simulink model "COMPTORQUE_Amato"  (R2018b)
settings: Solver=VariableStepAuto  StartTime=0.0  StopTime=10  RelTol=1e-3
values from neighbouring files (symbols this model uses):
  cond_init = [x1,x2,x3,x4,x5,x6]'    [Init.m]    (also in WS_regressor.mat = [0.523598775598 2.09439510239 -1.0471975512 1.57079632679 1.)
  Law = [kp, kd]    [Init.m]    (also in LAUNCH_Backstepping.m = [lambda, kd]; LAUNCH_Backstepping_adapt.m; LAUNCH_CToque.m; WS_regressor.mat = [500 50])
  param = param'    [Init.m]    (also in WS_regressor.mat = [1 1 1 1 1 1 0 1 1 1 3 3 ... (14 elements, 7x2)])
  pulsazione_circolare = 1    [Init.m]    (also in WS_regressor.mat)
  x0 = -1.5    [Init.m]    (also in WS_regressor.mat)
  y0 = 2    [Init.m]    (also in WS_regressor.mat)
undefined symbols (not defined in the file or in its folder): A_circolare
libraries: simulink x1
settings Model: Creator=AmatoPi  LastModifiedBy=Utente

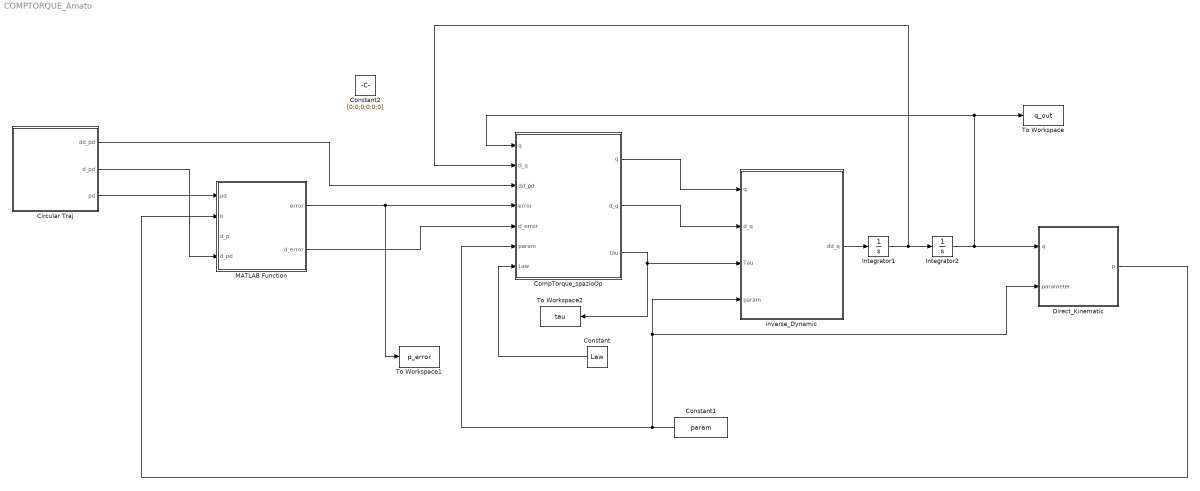
== system COMPTORQUE_Amato ==
  Circular Traj : Subsystem
  CompTorque_spazioOp : MATLAB Function  TreatAsAtomicUnit=on
  Constant : Constant  Value=Law
  Constant1 : Constant  Value=param
  Constant2 : Constant  Value=[0;0;0;0;0;0]
  Direct_Kinematic : MATLAB Function  TreatAsAtomicUnit=on
  Integrator1 : Integrator  InitialCondition=[0;0;0;0;0;0]
  Integrator2 : Integrator  InitialCondition=cond_init
  MATLAB Function : MATLAB Function  TreatAsAtomicUnit=on
  To Workspace : ToWorkspace  VariableName=q_out  SaveFormat=Structure With Time  SampleTime=-1
  To Workspace1 : ToWorkspace  VariableName=p_error  SaveFormat=Structure With Time  SampleTime=-1
  To Workspace2 : ToWorkspace  VariableName=tau  SaveFormat=Structure With Time  SampleTime=-1
  inverse_Dynamic : MATLAB Function  TreatAsAtomicUnit=on
  wires:
  CompTorque_spazioOp/2(d_q) -> inverse_Dynamic/2(d_q)
  CompTorque_spazioOp/1(q) -> inverse_Dynamic/1(q)
  inverse_Dynamic/1(dd_q) -> Integrator1/1
  Integrator1/1 -> CompTorque_spazioOp/2("d_q "), Integrator2/1
  Integrator2/1 -> CompTorque_spazioOp/1("q "), To Workspace/1, Direct_Kinematic/1(q)
  Constant/1 -> CompTorque_spazioOp/7(Law)
  Constant1/1 -> Direct_Kinematic/2(parameter), inverse_Dynamic/4(param), CompTorque_spazioOp/6(param)
  Circular Traj/3(pd) -> MATLAB Function/1(pd)
  Direct_Kinematic/1(p) -> MATLAB Function/2(p)
  MATLAB Function/1(error) -> To Workspace1/1, CompTorque_spazioOp/4(error)
  CompTorque_spazioOp/3(tau) -> To Workspace2/1, inverse_Dynamic/3(Tau)
  MATLAB Function/2(d_error) -> CompTorque_spazioOp/5(d_error)
  Circular Traj/2(d_pd) -> MATLAB Function/4(d_pd)
  Circular Traj/1(dd_pd) -> CompTorque_spazioOp/3(dd_pd)

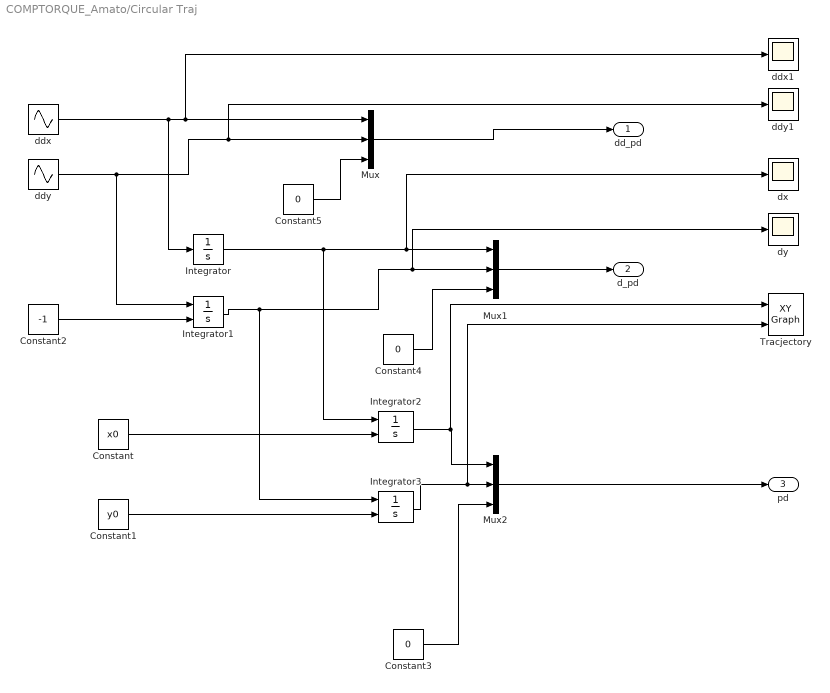
== system COMPTORQUE_Amato/Circular Traj ==
  Constant : Constant  Value=x0
  Constant1 : Constant  Value=y0
  Constant2 : Constant  Value=-1
  Constant3 : Constant  Value=0
  Constant4 : Constant  Value=0
  Constant5 : Constant  Value=0
  Integrator : Integrator
  Integrator1 : Integrator  InitialConditionSource=external
  Integrator2 : Integrator  InitialConditionSource=external
  Integrator3 : Integrator  InitialConditionSource=external
  Mux : Mux  Inputs=3
  Mux1 : Mux  Inputs=3
  Mux2 : Mux  Inputs=3
  Tracjectory : simulink/Sinks/XY Graph  xmin=xL  xmax=xR  ymin=yD  ymax=yU  st=-1
  ddx : Sin  Amplitude=A_circolare  Frequency=pulsazione_circolare  Phase=pi/2  SampleTime=0
  ddx1 : Scope
  ddy : Sin  Amplitude=A_circolare  Frequency=pulsazione_circolare  SampleTime=0
  ddy1 : Scope
  dx : Scope
  dy : Scope
  dd_pd : Outport
  d_pd : Outport  Port=2
  pd : Outport  Port=3
  wires:
  Mux/1 -> dd_pd/1
  ddx/1 -> Integrator/1, ddx1/1, Mux/1
  ddy/1 -> ddy1/1, Mux/2, Integrator1/1
  Mux1/1 -> d_pd/1
  Integrator2/1 -> Tracjectory/1, Mux2/1
  Mux2/1 -> pd/1
  Integrator/1 -> Integrator2/1, dx/1, Mux1/1
  Integrator3/1 -> Tracjectory/2, Mux2/2
  Integrator1/1 -> Integrator3/1, dy/1, Mux1/2
  Constant/1 -> Integrator2/2
  Constant1/1 -> Integrator3/2
  Constant2/1 -> Integrator1/2
  Constant3/1 -> Mux2/3
  Constant4/1 -> Mux1/3
  Constant5/1 -> Mux/3

== matlab function COMPTORQUE_Amato/CompTorque_spazioOp ==
  data: q input; q output; d_q output; d_q input; dd_pd input; tau output; error input; d_error input; param input; Law input
function [q,d_q,tau]  = CompTorque_Contro(q, d_q, dd_pd, error, d_error, param, Law)

    kp = Law(1).*eye(3);    
    kd = Law(2).*eye(3);
    
    [B,C,G] = Dinamica(param,q,d_q);
        
    J_hand = J_hand_fun(q);
    J_lessT = pinv(J_hand');
    
    d_J_hand = jacobian_derivative(q,d_q);
    
    Mx = J_lessT*B*pinv(J_hand);
    Hx = J_lessT*(C*d_q+G)-Mx*d_J_hand*d_q;
    F = Mx*(dd_pd + kd*d_error + kp*error) + Hx;
%     F = Mx*(dd_pd + kp*error) + Hx;
    tau = (J_hand')*F;

    
end

== matlab function COMPTORQUE_Amato/MATLAB Function ==
  data: pd input; error output; p input; d_p input; d_pd input; d_error output
function [error,d_error] = gen_error(pd,p, d_p, d_pd)
    
    p_now = p(6,1:3);

    error = pd-p_now';
    d_error = d_pd - pd;

end

== matlab function COMPTORQUE_Amato/inverse_Dynamic ==
  data: q input; dd_q output; d_q input; Tau input; param input
function dd_q = inverseDynamic(q, d_q, Tau, param)
    
    [B,C,G] = Dinamica(param,q,d_q);

    tot = Tau - C*d_q - G;    
    dd_q = B\(tot);

end

== matlab function COMPTORQUE_Amato/Direct_Kinematic ==
  data: q input; p output; parameter input
function p = DirectK(q,parameter)

	[p,com,head] = Direct_Kinematics(parameter,q);
    
    

end
